simulink model "nonlinear_ball_and_beam_simulink"  (R2022a)
settings: Solver=VariableStepAuto  StartTime=0.0  StopTime=100.0  RelTol=1e-3
values from neighbouring files (symbols this model uses):
  a22 = - ganho_angulo_antigo/(Jv + mb * delta^2 )    (= -1.39833231431)    [ball_and_beam_pfc.m]
  a23 = -(( mb * Jv *g + (mb^2 )*g * delta^2 )/((Jv + mb*delta^2)^2))    (= -10.2378061844)    [ball_and_beam_pfc.m]
  a41 = -5*g/7    (= -7)    [ball_and_beam_pfc.m]
  b21 = ganho_entrada_antigo /(Jv + mb * delta^2 )    (= 3.67687876407)    [ball_and_beam_pfc.m]
  d = 0.12    [ball_and_beam_pfc.m]    (also in nonlinear_ball_and_beam.m)
  g = 9.8    [ball_and_beam_pfc.m]    (also in nonlinear_ball_and_beam.m)
  Jv = (1/2) * mv * L^2    (= 0.058703125)    [ball_and_beam_pfc.m]    (also in nonlinear_ball_and_beam.m)
  Kg = 14    [ball_and_beam_pfc.m]    (also in nonlinear_ball_and_beam.m)
  Ki = 0.00767    [ball_and_beam_pfc.m]    (also in nonlinear_ball_and_beam.m)
  L = 0.425    [ball_and_beam_pfc.m]    (also in nonlinear_ball_and_beam.m)
  mb = 0.064    [ball_and_beam_pfc.m]    (also in nonlinear_ball_and_beam.m)
  mv = 0.65    [ball_and_beam_pfc.m]    (also in nonlinear_ball_and_beam.m)
  N_total = N_motor + N_gearbox    (= 1.54)    [ball_and_beam_pfc.m]    (also in nonlinear_ball_and_beam.m)
  Rm = 2.6    [ball_and_beam_pfc.m]    (also in nonlinear_ball_and_beam.m)
libraries: slpidlib x1
settings Model: Creator=Notebook_Artur  LastModifiedBy=Notebook_Artur

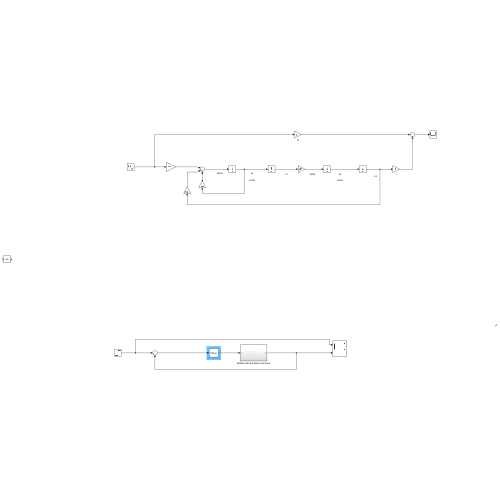
[thumbnail: Simulink's stored preview of the top-level diagram]
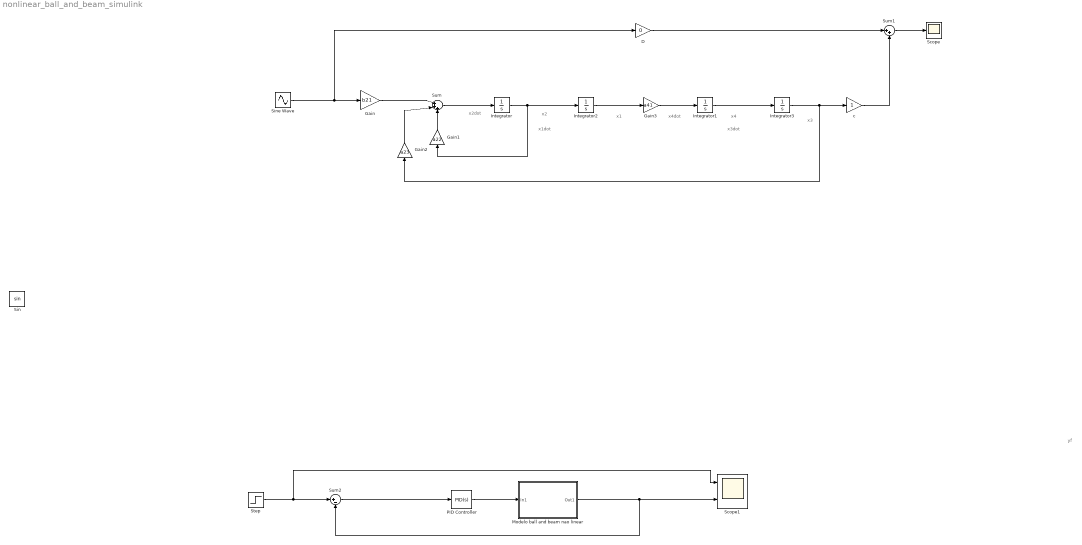
== system nonlinear_ball_and_beam_simulink ==
  note: yf
  note: x1
  note: x3
  note: x1dot
  note: x2
  note: x3dot
  note: x4
  note: x4dot
  note: x2dot
  D : Gain  Gain=0
  Gain : Gain  Gain=b21
  Gain1 : Gain  Gain=a22
  Gain2 : Gain  Gain=a23
  Gain3 : Gain  Gain=a41
  Integrator{,1..3} (4 alike) : Integrator
  Modelo ball and beam nao linear : Subsystem
  PID Controller : slpidlib/PID Controller  Controller=PID  Form=Parallel  TimeDomain=Continuous-time  UseExternalTs=off  SampleTime=-1  IntegratorMethod=Forward Euler  FilterMethod=Forward Euler  ControllerParametersSource=internal  P=-2.13960854480505  I=-0.137623555421651  UseKiTs=off  D=-6.18126043354076  N=9.58491119024195  UseFilter=on  TunerSelectOption=Transfer Function Based (PID Tuner App)  InitialConditionSource=internal  InitialConditionForIntegrator=0  InitialConditionForFilter=0  DifferentiatorICPrevScaledInput=0  ExternalReset=none  TrackingMode=off  Kt=1  LimitOutput=off  SatLimitsSource=internal  UpperSaturationLimit=inf  LowerSaturationLimit=-inf  LinearizeAsGain=on  AntiWindupMode=none  Kb=1  POutMin=[]  POutMax=[]  IOutMin=[]  IOutMax=[]  DOutMin=[]  DOutMax=[]  NOutMin=[]  NOutMax=[]  SumOutMin=[]  SumOutMax=[]  SaturationOutMin=[]  SaturationOutMax=[]  PParamMin=[]  PParamMax=[]  IParamMin=[]  IParamMax=[]  DParamMin=[]  DParamMax=[]  NParamMin=[]  NParamMax=[]  KbParamMin=[]  KbParamMax=[]  KtParamMin=[]  KtParamMax=[]  KbOutMin=[]  KbOutMax=[]  KtOutMin=[]  KtOutMax=[]  IntegratorOutMin=[]  IntegratorOutMax=[]  FilterOutMin=[]  FilterOutMax=[]  SumI1OutMin=[]  SumI1OutMax=[]  SumI2OutMin=[]  SumI2OutMax=[]  SumI3OutMin=[]  SumI3OutMax=[]  SumI4OutMin=[]  SumI4OutMax=[]  SumDOutMin=[]  SumDOutMax=[]  DifferentiatorOutMin=[]  DifferentiatorOutMax=[]  FilterDiffOutCoefMin=[]  FilterDiffOutCoefMax=[]  ReciprocalOutMin=[]  ReciprocalOutMax=[]  SumDenOutMin=[]  SumDenOutMax=[]  SumNumOutMin=[]  SumNumOutMax=[]  DivideOutMin=[]  DivideOutMax=[]  UdiffTsProdOutMin=[]  UdiffTsProdOutMax=[]  NTsProdOutMin=[]  NTsProdOutMax=[]  UintegralTsProdOutMin=[]  UintegralTsProdOutMax=[]  UngainTsProdOutMin=[]  UngainTsProdOutMax=[]  IntegratorContinuousStateAttributes=''  IntegratorStateMustResolveToSignalObject=off  IntegratorRTWStateStorageClass=Auto  FilterContinuousStateAttributes=''  FilterStateMustResolveToSignalObject=off  FilterRTWStateStorageClass=Auto  ParallelPVariant=InternalParameters  IdealPVariant=Disabled  IVariant=InternalParameters  DVariant=InternalParameters  IntegratorVariant=Continuous  SatVariant=Disabled  AWVariant=Passthrough  PCopyVariant=Disabled  TRVariant=Disabled  FdbkBlocksVariant=Forward  IdealPFdbkVariant=Disabled  SatFdbkVariant=Disabled  DerivativeFilterVariant=ContFilter  NVariant=InternalParameters  NCopyVariant=Disabled  FilterICVariant=InternalICsFilter  IntegratorICVariant=InternalICs  ExternalResetVariant=Disabled  TRSumVariant=Passthrough  SumFdbkVariant=Disabled  SumVariant=Sum_PID  TsampFilterVariant=InternalTs  TsampNgainVariant=Passthrough  TsampIntegralVariant=Passthrough  ExternalSaturationOutDataTypeStr=Inherit: Same as second input  aMode=0
  Scope : Scope
  Scope1 : Scope  NumInputPorts=2
  Sin : Trigonometry
  Sine Wave : Sin  SampleTime=0
  Step : Step  SampleTime=0
  Sum : Sum  Inputs=|+++
  Sum1 : Sum  Inputs=|++
  Sum2 : Sum  Inputs=|+-
  c : Gain
  wires:
  Sine Wave/1 -> D/1, Gain/1
  Integrator/1 -> Gain1/1, Integrator2/1
  Gain/1 -> Sum/1
  Gain2/1 -> Sum/2
  Gain1/1 -> Sum/3
  Sum/1 -> Integrator/1
  Integrator3/1 -> c/1, Gain2/1
  Gain3/1 -> Integrator1/1
  Integrator2/1 -> Gain3/1
  Integrator1/1 -> Integrator3/1
  c/1 -> Sum1/2
  D/1 -> Sum1/1
  Sum1/1 -> Scope/1
  Step/1 -> Sum2/1, Scope1/1
  Modelo ball and beam nao linear/1(Out1) -> Sum2/2, Scope1/2
  PID Controller/1 -> Modelo ball and beam nao linear/1(In1)
  Sum2/1 -> PID Controller/1

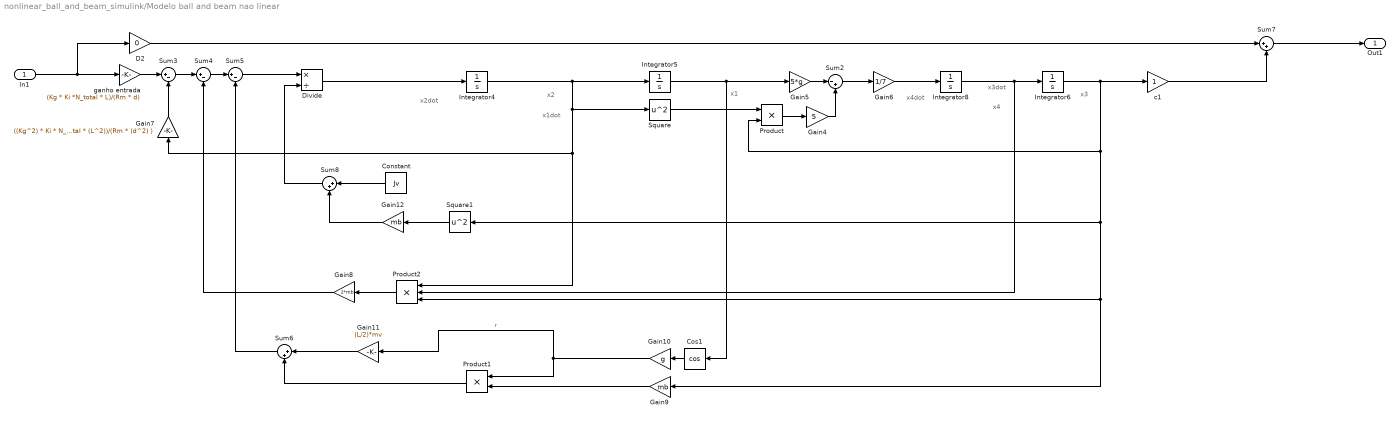
== system nonlinear_ball_and_beam_simulink/Modelo ball and beam nao linear ==
  note: x3
  note: x3dot
  note: x4
  note: x4dot
  note: x1
  note: x1dot
  note: x2dot
  note: x2
  In1 : Inport
  Constant : Constant  Value=Jv
  Cos1 : Trigonometry  Operator=cos
  D2 : Gain  Gain=0
  Divide : Product  Inputs=*/
  Gain10 : Gain  Gain=g
  Gain11 : Gain  Gain=(L/2)*mv
  Gain12 : Gain  Gain=mb
  Gain4 : Gain  Gain=5
  Gain5 : Gain  Gain=5*g
  Gain6 : Gain  Gain=1/7
  Gain7 : Gain  Gain=((Kg^2) * Ki * N_total * (L^2))/(Rm * (d^2) )
  Gain8 : Gain  Gain=2*mb
  Gain9 : Gain  Gain=mb
  Integrator{4..6,8} (4 alike) : Integrator
  Product : Product
  Product1 : Product
  Product2 : Product  Inputs=3
  Square : Math  Operator=square
  Square1 : Math  Operator=square
  Sum2 : Sum  Inputs=|-+
  Sum3 : Sum  Inputs=|+-
  Sum4 : Sum  Inputs=|+-
  Sum5 : Sum  Inputs=|+-
  Sum6 : Sum  Inputs=|++
  Sum7 : Sum  Inputs=|++
  Sum8 : Sum  Inputs=|++
  c1 : Gain
  ganho entrada : Gain  Gain=(Kg * Ki *N_total * L)/(Rm * d)
  Out1 : Outport
  wires:
  Integrator8/1 -> Product2/2, Integrator6/1
  Integrator4/1 -> Product2/1, Gain7/1, Square/1, Integrator5/1
  c1/1 -> Sum7/2
  Integrator5/1 -> Cos1/1, Gain5/1
  Sum6/1 -> Sum5/2
  Sum3/1 -> Sum4/1
  Sum2/1 -> Gain6/1
  Gain10/1 -> Product1/1, Gain11/1  "r"
  Square/1 -> Product/1
  Integrator6/1 -> c1/1, Square1/1, Gain9/1, Product2/3, Product/2
  Gain11/1 -> Sum6/1
  Gain12/1 -> Sum8/2
  In1/1 -> D2/1, ganho entrada/1
  Gain5/1 -> Sum2/1
  D2/1 -> Sum7/1
  Gain6/1 -> Integrator8/1
  Sum4/1 -> Sum5/1
  Gain4/1 -> Sum2/2
  Gain7/1 -> Sum3/2
  Sum5/1 -> Divide/1
  ganho entrada/1 -> Sum3/1
  Gain9/1 -> Product1/2
  Cos1/1 -> Gain10/1
  Gain8/1 -> Sum4/2
  Divide/1 -> Integrator4/1
  Product2/1 -> Gain8/1
  Product/1 -> Gain4/1
  Square1/1 -> Gain12/1
  Sum8/1 -> Divide/2
  Product1/1 -> Sum6/2
  Constant/1 -> Sum8/1
  Sum7/1 -> Out1/1
